simulink model "mvt"  (R2024b)
settings: Solver=VariableStepAuto  StartTime=0.0  StopTime=10.0  RelTol=1e-3
libraries: fl_lib x22, nesl_utility x12

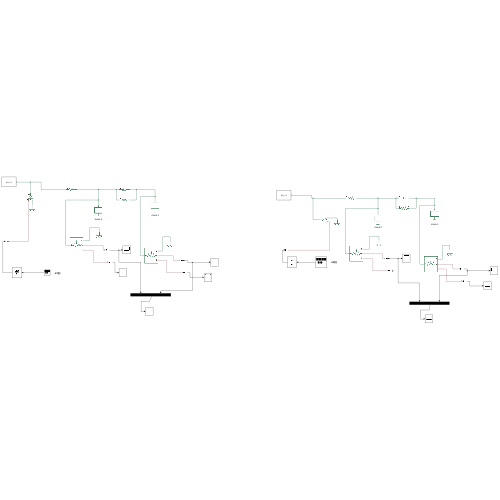
[thumbnail: Simulink's stored preview of the top-level diagram]
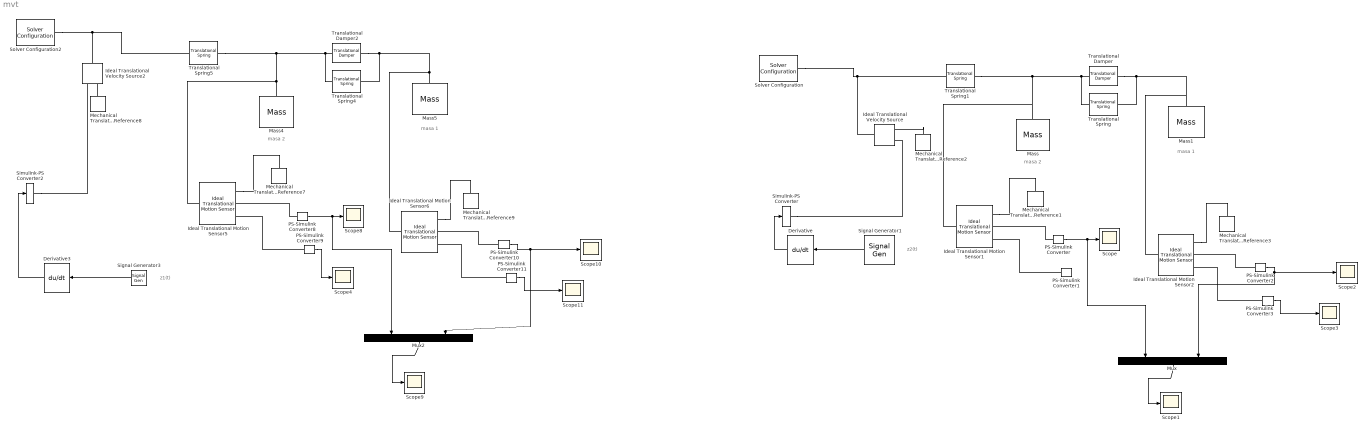
== system mvt ==
  note: masa 1
  note: z2(t)
  note: masa 2
  note: masa 1
  note: masa 2
  note: z1(t)
  Derivative : Derivative
  Derivative3 : Derivative
  Ideal Translational Motion Sensor{1..2,5..6} (4 alike) : fl_lib/Mechanical/Mechanical Sensors/Ideal Translational Motion Sensor  reference=foundation.enum.MeasurementReference.difference  acceleration_port=false  velocity_port=true  position_port=true  offset=0 m
  Ideal Translational Velocity Source : fl_lib/Mechanical/Mechanical Sources/Ideal Translational Velocity Source
  Ideal Translational Velocity Source2 : fl_lib/Mechanical/Mechanical Sources/Ideal Translational Velocity Source
  Mass : fl_lib/Mechanical/Translational Elements/Mass  mass=59 kg  num_ports=foundation.enum.numPorts2.one  v_specify=on  v_priority=High  v=1 m/s  v_nominal_specify=off  v_nominal_value=1  v_nominal_unit=m/s  f_specify=off  f_priority=None  f=0 N  f_nominal_specify=off  f_nominal_value=1  f_nominal_unit=N
  Mass1 : fl_lib/Mechanical/Translational Elements/Mass  mass=290 kg  num_ports=foundation.enum.numPorts2.one  v_specify=on  v_priority=High  v=1 m/s  v_nominal_specify=off  v_nominal_value=1  v_nominal_unit=m/s  f_specify=off  f_priority=None  f=0 N  f_nominal_specify=off  f_nominal_value=1  f_nominal_unit=N
  Mass4 : fl_lib/Mechanical/Translational Elements/Mass  mass=59 kg  num_ports=foundation.enum.numPorts2.one  v_specify=on  v_priority=High  v=1 m/s  v_nominal_specify=off  v_nominal_value=1  v_nominal_unit=m/s  f_specify=off  f_priority=None  f=0 N  f_nominal_specify=off  f_nominal_value=1  f_nominal_unit=N
  Mass5 : fl_lib/Mechanical/Translational Elements/Mass  mass=290 kg  num_ports=foundation.enum.numPorts2.one  v_specify=on  v_priority=High  v=1 m/s  v_nominal_specify=off  v_nominal_value=1  v_nominal_unit=m/s  f_specify=off  f_priority=None  f=0 N  f_nominal_specify=off  f_nominal_value=1  f_nominal_unit=N
  Mechanical Translational Reference{1..3,7..9} (6 alike) : fl_lib/Mechanical/Translational Elements/Mechanical Translational Reference
  Mux : Mux  Inputs=2
  Mux2 : Mux  Inputs=2
  PS-Simulink Converter{,1..3,8..11} (8 alike) : nesl_utility/PS-Simulink Converter  PhysicalDomain=network_engine_domain  SubClassName=ps_output  LeftPortType=input  RightPortType=output  PseudoPeriodic=off  Frequencies=[]  VectorFormat=inherit  Unit=inherit  AffineConversion=off
  Scope{,1..4,8..11} (9 alike) : Scope
  Signal Generator1 : SignalGenerator  Amplitude=0.05  Frequency=20*pi  Units=rad/sec
  Signal Generator3 : SignalGenerator  Amplitude=0.05  Frequency=0.5*pi  Units=rad/sec
  Simulink-PS Converter : nesl_utility/Simulink-PS Converter  PhysicalDomain=network_engine_domain  SubClassName=ps_input  LeftPortType=input  RightPortType=output  PseudoPeriodic=off  Frequencies=[]  NoiseDistribution=none  NoiseParameters=[]  Unit=1  AffineConversion=off  FilteringAndDerivatives=provide  SimscapeFilterOrder=1  InputFilterTimeConstant=0.001  UdotUserProvided=0
  Simulink-PS Converter2 : nesl_utility/Simulink-PS Converter  PhysicalDomain=network_engine_domain  SubClassName=ps_input  LeftPortType=input  RightPortType=output  PseudoPeriodic=off  Frequencies=[]  NoiseDistribution=none  NoiseParameters=[]  Unit=1  AffineConversion=off  FilteringAndDerivatives=provide  SimscapeFilterOrder=1  InputFilterTimeConstant=0.001  UdotUserProvided=0
  Solver Configuration : nesl_utility/Solver Configuration  PhysicalDomain=network_engine_domain  SubClassName=solver  LeftPortType=input  RightPortType=generic  Tones=[]  Harmonics=[]  SimulateNoise=off  Profile=off  UseLocalSampling=off  EnableSwitchedLinearOptims=on  FrequencyDomain=off  UseCCode=off  RelTol=0.001  AbsTol=0.001  MinStep=1e-09  ToWorkspace=off  RevertToSquareIcSolve=off  NumHomotopyIterations=100  PhasorMode=off  PhasorModeNumHarmonics=1  ConsistencySolver=NEWTON_XTOL_AFTER_FTOL  IndexReductionMethod=DerivativeReplacement  DoDC=off  ResidualTolerance=1e-09  ConsistencyTolSource=GLOBAL  ConsistencyAbsTol=0.001  ConsistencyRelTol=0.001  ConsistencyTolFactor=0.001  UseLocalSolver=off  LocalSolverChoice=NE_BACKWARD_EULER_ADVANCER  ResolveIndetEquations=on  FunctionEvalNumThread=1  LocalSolverSampleTime=0.001  DoFixedCost=off  MaxNonlinIter=3  MaxModeIter=2  ComputeImpulses=off  ImpulseIterations=2  LinearAlgebra=auto  LinearAlgebraNumThread=0  EquationFormulation=NE_TIME_EF  DelaysMemoryBudget=1024  AutomaticFiltering=on  FilteringTimeConstant=0.001  PartitionStorageMethod=AS_NEEDED  PartitionMemoryBudget=1024  PartitionMethod=ROBUST  MultibodyUseLocalSolver=off  MultibodyLocalSolverChoice=ODE1  MultibodyLocalSolverSampleTime=0.001
  Solver Configuration2 : nesl_utility/Solver Configuration  PhysicalDomain=network_engine_domain  SubClassName=solver  LeftPortType=input  RightPortType=generic  Tones=[]  Harmonics=[]  SimulateNoise=off  Profile=off  UseLocalSampling=off  EnableSwitchedLinearOptims=on  FrequencyDomain=off  UseCCode=off  RelTol=0.001  AbsTol=0.001  MinStep=1e-09  ToWorkspace=off  RevertToSquareIcSolve=off  NumHomotopyIterations=100  PhasorMode=off  PhasorModeNumHarmonics=1  ConsistencySolver=NEWTON_XTOL_AFTER_FTOL  IndexReductionMethod=DerivativeReplacement  DoDC=off  ResidualTolerance=1e-09  ConsistencyTolSource=GLOBAL  ConsistencyAbsTol=0.001  ConsistencyRelTol=0.001  ConsistencyTolFactor=0.001  UseLocalSolver=off  LocalSolverChoice=NE_BACKWARD_EULER_ADVANCER  ResolveIndetEquations=on  FunctionEvalNumThread=1  LocalSolverSampleTime=0.001  DoFixedCost=off  MaxNonlinIter=3  MaxModeIter=2  ComputeImpulses=off  ImpulseIterations=2  LinearAlgebra=auto  LinearAlgebraNumThread=0  EquationFormulation=NE_TIME_EF  DelaysMemoryBudget=1024  AutomaticFiltering=on  FilteringTimeConstant=0.001  PartitionStorageMethod=AS_NEEDED  PartitionMemoryBudget=1024  PartitionMethod=ROBUST  MultibodyUseLocalSolver=off  MultibodyLocalSolverChoice=ODE1  MultibodyLocalSolverSampleTime=0.001
  Translational Damper : fl_lib/Mechanical/Translational Elements/Translational Damper  D=1000 N*s/m  v_specify=off  v_priority=None  v=0 m/s  v_nominal_specify=off  v_nominal_value=1  v_nominal_unit=m/s  f_specify=off  f_priority=None  f=0 N  f_nominal_specify=off  f_nominal_value=1  f_nominal_unit=N
  Translational Damper2 : fl_lib/Mechanical/Translational Elements/Translational Damper  D=1000 N*s/m  v_specify=off  v_priority=None  v=0 m/s  v_nominal_specify=off  v_nominal_value=1  v_nominal_unit=m/s  f_specify=off  f_priority=None  f=0 N  f_nominal_specify=off  f_nominal_value=1  f_nominal_unit=N
  Translational Spring : fl_lib/Mechanical/Translational Elements/Translational Spring  spr_rate=16182 N/m  v_specify=off  v_priority=None  v=0 m/s  v_nominal_specify=off  v_nominal_value=1  v_nominal_unit=m/s  f_specify=off  f_priority=None  f=0 N  f_nominal_specify=off  f_nominal_value=1  f_nominal_unit=N  x_specify=off  x_priority=High  x=0 m  x_nominal_specify=off  x_nominal_value=1  x_nominal_unit=m
  Translational Spring1 : fl_lib/Mechanical/Translational Elements/Translational Spring  spr_rate="19000  N/m"  v_specify=off  v_priority=None  v=0 m/s  v_nominal_specify=off  v_nominal_value=1  v_nominal_unit=m/s  f_specify=off  f_priority=None  f=0 N  f_nominal_specify=off  f_nominal_value=1  f_nominal_unit=N  x_specify=off  x_priority=High  x=0 m  x_nominal_specify=off  x_nominal_value=1  x_nominal_unit=m
  Translational Spring4 : fl_lib/Mechanical/Translational Elements/Translational Spring  spr_rate=16182 N/m  v_specify=off  v_priority=None  v=0 m/s  v_nominal_specify=off  v_nominal_value=1  v_nominal_unit=m/s  f_specify=off  f_priority=None  f=0 N  f_nominal_specify=off  f_nominal_value=1  f_nominal_unit=N  x_specify=off  x_priority=High  x=0 m  x_nominal_specify=off  x_nominal_value=1  x_nominal_unit=m
  Translational Spring5 : fl_lib/Mechanical/Translational Elements/Translational Spring  spr_rate="19000  N/m"  v_specify=off  v_priority=None  v=0 m/s  v_nominal_specify=off  v_nominal_value=1  v_nominal_unit=m/s  f_specify=off  f_priority=None  f=0 N  f_nominal_specify=off  f_nominal_value=1  f_nominal_unit=N  x_specify=off  x_priority=High  x=0 m  x_nominal_specify=off  x_nominal_value=1  x_nominal_unit=m
  wires:
  Derivative/1 -> Simulink-PS Converter/1
  Mux/1 -> Scope1/1
  PS-Simulink Converter/1 -> Mux/1, Scope/1
  PS-Simulink Converter2/1 -> Mux/2, Scope2/1
  PS-Simulink Converter3/1 -> Scope3/1
  PS-Simulink Converter8/1 -> Mux2/1, Scope8/1
  PS-Simulink Converter9/1 -> Scope4/1
  Derivative3/1 -> Simulink-PS Converter2/1
  PS-Simulink Converter10/1 -> Mux2/2, Scope10/1
  PS-Simulink Converter11/1 -> Scope11/1
  Mux2/1 -> Scope9/1
  Signal Generator1/1 -> Derivative/1
  Signal Generator3/1 -> Derivative3/1
  connections:
  PS-Simulink Converter/LConn1 -- Ideal Translational Motion Sensor1/RConn2
  PS-Simulink Converter1/LConn1 -- Ideal Translational Motion Sensor1/RConn3
  Ideal Translational Motion Sensor1/RConn1 -- Mechanical Translational Reference1/LConn1
  PS-Simulink Converter2/LConn1 -- Ideal Translational Motion Sensor2/RConn2
  PS-Simulink Converter3/LConn1 -- Ideal Translational Motion Sensor2/RConn3
  Mechanical Translational Reference2/LConn1 -- Ideal Translational Velocity Source/RConn2
  Ideal Translational Motion Sensor2/RConn1 -- Mechanical Translational Reference3/LConn1
  Solver Configuration/RConn1 -- Ideal Translational Velocity Source/LConn1 -- Translational Spring1/LConn1
  Simulink-PS Converter/RConn1 -- Ideal Translational Velocity Source/RConn1
  Translational Damper/RConn1 -- Ideal Translational Motion Sensor2/LConn1 -- Mass1/LConn1 -- Translational Spring/RConn1
  Translational Damper/LConn1 -- Ideal Translational Motion Sensor1/LConn1 -- Mass/LConn1 -- Translational Spring1/RConn1 -- Translational Spring/LConn1
  Mass5/LConn1 -- Ideal Translational Motion Sensor6/LConn1 -- Translational Damper2/RConn1 -- Translational Spring4/RConn1
  Mass4/LConn1 -- Ideal Translational Motion Sensor5/LConn1 -- Translational Damper2/LConn1 -- Translational Spring4/LConn1 -- Translational Spring5/RConn1
  Simulink-PS Converter2/RConn1 -- Ideal Translational Velocity Source2/RConn1
  PS-Simulink Converter8/LConn1 -- Ideal Translational Motion Sensor5/RConn2
  Ideal Translational Motion Sensor6/RConn1 -- Mechanical Translational Reference9/LConn1
  Mechanical Translational Reference8/LConn1 -- Ideal Translational Velocity Source2/RConn2
  PS-Simulink Converter9/LConn1 -- Ideal Translational Motion Sensor5/RConn3
  PS-Simulink Converter10/LConn1 -- Ideal Translational Motion Sensor6/RConn2
  Ideal Translational Motion Sensor5/RConn1 -- Mechanical Translational Reference7/LConn1
  PS-Simulink Converter11/LConn1 -- Ideal Translational Motion Sensor6/RConn3
  Solver Configuration2/RConn1 -- Ideal Translational Velocity Source2/LConn1 -- Translational Spring5/LConn1
